simulink model "model_sim_CHB5_36pulse_23b"  (R2023b)
settings: Solver=FixedStepAuto  StartTime=0.0  StopTime=10  RelTol=1e-3
InitFcn:
  | sysinit
values from neighbouring files (symbols this model uses):
  C = 0.03    [sysinit.m]
  C_f = 0.625e-6    (= 6.25e-07)    [sysinit.m]
  L = 0.004    [sysinit.m]
  L_f = 3e-6    (= 3e-06)    [sysinit.m]
  R = 1.2    [sysinit.m]
  R_f = 1.5    [sysinit.m]
  st = 5e-7    (= 5e-07)    [sysinit.m]
libraries: spsSeriesRLCBranchLib x142, spsDiodeLib x60, spsIGBTLib x48, spsCurrentMeasurementLib x22, spsRMSLib x9, spsVoltageMeasurementLib x9, spsThreePhaseVIMeasurementLib x7, spsZigzagPhaseShiftingTransformerLib x6, spsUniversalBridgeLib x6, spsOnDelayLib x6, simulink x5, spsDistributedParametersLineLib x1
(part 3 of 3)

== system model_sim_CHB5_36pulse_23b/Subsystem/IGCT5 ==
  PWM : Inport
  Current Measurement1 : spsCurrentMeasurementLib/Current Measurement  PhasorSimulation=off  OutputType=Complex  PSBequivalent=0
  Demux : Demux
  Diode{1..3,6,8} (5 alike) : spsDiodeLib/Diode  Ron=DIODE.rF  Lon=0  Vf=DIODE.VF0  IC=0  UseSnubber=off  Rs=500  Cs=250e-9  Measurements=on
  IGBT{,1..3} (4 alike) : spsIGBTLib/IGBT  Ron=IGCT.rT  Lon=0  Vf=IGCT.VT0  Tf=1e-6  Tt=2e-6  IC=0  Rs=1e5  Cs=inf  Measurements=on
  Series RLC Branch1 : spsSeriesRLCBranchLib/Series RLC Branch  LConnTagsString=__new0  RConnTagsString=__new0  BranchType=RL  Resistance=1e-5  Inductance=3.0E-6  SetiL0=off  InitialCurrent=0  Capacitance=1e-6  Setx0=off  InitialVoltage=0  Measurements=None
  Series RLC Branch10 : spsSeriesRLCBranchLib/Series RLC Branch  LConnTagsString=__new0  RConnTagsString=__new0  BranchType=L  Resistance=1  Inductance=0.4e-6  SetiL0=off  InitialCurrent=0  Capacitance=1e-6  Setx0=off  InitialVoltage=0  Measurements=None
  Series RLC Branch12 : spsSeriesRLCBranchLib/Series RLC Branch  LConnTagsString=__new0  RConnTagsString=__new0  BranchType=RL  Resistance=1e-5  Inductance=1E-9  SetiL0=off  InitialCurrent=0  Capacitance=1e-6  Setx0=off  InitialVoltage=0  Measurements=None
  Series RLC Branch14 : spsSeriesRLCBranchLib/Series RLC Branch  LConnTagsString=__new0  RConnTagsString=__new0  BranchType=L  Resistance=1  Inductance=1E-7  SetiL0=off  InitialCurrent=0  Capacitance=1e-6  Setx0=off  InitialVoltage=0  Measurements=None
  Series RLC Branch2 : spsSeriesRLCBranchLib/Series RLC Branch  LConnTagsString=__new0  RConnTagsString=__new0  BranchType=RC  Resistance=1e-5  Inductance=20e-6  SetiL0=off  InitialCurrent=0  Capacitance=17e-6  Setx0=off  InitialVoltage=0  Measurements=None
  Series RLC Branch3 : spsSeriesRLCBranchLib/Series RLC Branch  LConnTagsString=__new0  RConnTagsString=__new0  BranchType=RL  Resistance=1e-5  Inductance=1E-9  SetiL0=off  InitialCurrent=0  Capacitance=1e-6  Setx0=off  InitialVoltage=0  Measurements=None
  Series RLC Branch5 : spsSeriesRLCBranchLib/Series RLC Branch  LConnTagsString=__new0  RConnTagsString=__new0  BranchType=L  Resistance=1  Inductance=1E-7  SetiL0=off  InitialCurrent=0  Capacitance=1e-6  Setx0=off  InitialVoltage=0  Measurements=None
  Series RLC Branch7 : spsSeriesRLCBranchLib/Series RLC Branch  LConnTagsString=__new0  RConnTagsString=__new0  BranchType=RL  Resistance=0.6  Inductance=1e-6  SetiL0=off  InitialCurrent=0  Capacitance=1e-6  Setx0=off  InitialVoltage=0  Measurements=None
  Series RLC Branch9 : spsSeriesRLCBranchLib/Series RLC Branch  LConnTagsString=__new0  RConnTagsString=__new0  BranchType=L  Resistance=1  Inductance=0.4e-6  SetiL0=off  InitialCurrent=0  Capacitance=1e-6  Setx0=off  InitialVoltage=0  Measurements=None
  Terminator{,1..9} (10 alike) : Terminator
  Udc+ : PMIOPort  Side=Left
  udc- : PMIOPort  Port=2  Side=Left
  p1 : PMIOPort  Port=3  Side=Right
  p2 : PMIOPort  Port=4  Side=Right
  wires:
  Diode3/1 -> Terminator9/1
  IGBT3/1 -> Terminator5/1
  [n1] -> IGBT3/1
  IGBT1/1 -> Terminator4/1
  IGBT2/1 -> Terminator3/1
  IGBT/1 -> Terminator2/1
  [n2] -> IGBT1/1
  [p1] -> IGBT2/1
  Current Measurement1/1 -> Terminator/1
  Diode2/1 -> Terminator8/1
  [p2] -> IGBT/1
  Diode8/1 -> Terminator7/1
  Diode1/1 -> Terminator6/1
  Diode6/1 -> Terminator1/1
  Demux/3 -> [n2]
  PWM/1 -> Demux/1
  Demux/1 -> [p2]
  Demux/2 -> [p1]
  Demux/4 -> [n1]
  connections:
  Series RLC Branch10/LConn1 -- udc-/RConn1
  Series RLC Branch9/LConn1 -- Udc+/RConn1
  Diode6/RConn1 -- Series RLC Branch7/RConn1 -- Series RLC Branch2/LConn1
  Current Measurement1/LConn1 -- Series RLC Branch1/RConn1 -- Series RLC Branch3/LConn1 -- Series RLC Branch12/LConn1
  IGBT3/RConn1 -- Series RLC Branch14/RConn1 -- Diode3/LConn1
  Series RLC Branch3/RConn1 -- IGBT/LConn1 -- Diode8/RConn1
  IGBT1/RConn1 -- Series RLC Branch5/RConn1 -- Diode1/LConn1
  Current Measurement1/RConn1 -- Diode6/LConn1
  Diode2/RConn1 -- Series RLC Branch12/RConn1 -- IGBT2/LConn1
  Diode2/LConn1 -- p1/RConn1 -- IGBT3/LConn1 -- IGBT2/RConn1 -- Diode3/RConn1
  Series RLC Branch5/LConn1 -- Series RLC Branch14/LConn1 -- Series RLC Branch10/RConn1 -- Series RLC Branch2/RConn1
  Series RLC Branch1/LConn1 -- Series RLC Branch7/LConn1 -- Series RLC Branch9/RConn1
  IGBT1/LConn1 -- p2/RConn1 -- Diode8/LConn1 -- IGBT/RConn1 -- Diode1/RConn1

== system model_sim_CHB5_36pulse_23b/Subsystem/IGCT6 ==
  PWM : Inport
  Current Measurement1 : spsCurrentMeasurementLib/Current Measurement  PhasorSimulation=off  OutputType=Complex  PSBequivalent=0
  Demux : Demux
  Diode{1..3,6,8} (5 alike) : spsDiodeLib/Diode  Ron=DIODE.rF  Lon=0  Vf=DIODE.VF0  IC=0  UseSnubber=off  Rs=500  Cs=250e-9  Measurements=on
  IGBT{,1..3} (4 alike) : spsIGBTLib/IGBT  Ron=IGCT.rT  Lon=0  Vf=IGCT.VT0  Tf=1e-6  Tt=2e-6  IC=0  Rs=1e5  Cs=inf  Measurements=on
  Series RLC Branch1 : spsSeriesRLCBranchLib/Series RLC Branch  LConnTagsString=__new0  RConnTagsString=__new0  BranchType=RL  Resistance=1e-5  Inductance=3.0E-6  SetiL0=off  InitialCurrent=0  Capacitance=1e-6  Setx0=off  InitialVoltage=0  Measurements=None
  Series RLC Branch10 : spsSeriesRLCBranchLib/Series RLC Branch  LConnTagsString=__new0  RConnTagsString=__new0  BranchType=L  Resistance=1  Inductance=0.4e-6  SetiL0=off  InitialCurrent=0  Capacitance=1e-6  Setx0=off  InitialVoltage=0  Measurements=None
  Series RLC Branch12 : spsSeriesRLCBranchLib/Series RLC Branch  LConnTagsString=__new0  RConnTagsString=__new0  BranchType=RL  Resistance=1e-5  Inductance=1E-9  SetiL0=off  InitialCurrent=0  Capacitance=1e-6  Setx0=off  InitialVoltage=0  Measurements=None
  Series RLC Branch14 : spsSeriesRLCBranchLib/Series RLC Branch  LConnTagsString=__new0  RConnTagsString=__new0  BranchType=L  Resistance=1  Inductance=1E-7  SetiL0=off  InitialCurrent=0  Capacitance=1e-6  Setx0=off  InitialVoltage=0  Measurements=None
  Series RLC Branch2 : spsSeriesRLCBranchLib/Series RLC Branch  LConnTagsString=__new0  RConnTagsString=__new0  BranchType=RC  Resistance=1e-5  Inductance=20e-6  SetiL0=off  InitialCurrent=0  Capacitance=17e-6  Setx0=off  InitialVoltage=0  Measurements=None
  Series RLC Branch3 : spsSeriesRLCBranchLib/Series RLC Branch  LConnTagsString=__new0  RConnTagsString=__new0  BranchType=RL  Resistance=1e-5  Inductance=1E-9  SetiL0=off  InitialCurrent=0  Capacitance=1e-6  Setx0=off  InitialVoltage=0  Measurements=None
  Series RLC Branch5 : spsSeriesRLCBranchLib/Series RLC Branch  LConnTagsString=__new0  RConnTagsString=__new0  BranchType=L  Resistance=1  Inductance=1E-7  SetiL0=off  InitialCurrent=0  Capacitance=1e-6  Setx0=off  InitialVoltage=0  Measurements=None
  Series RLC Branch7 : spsSeriesRLCBranchLib/Series RLC Branch  LConnTagsString=__new0  RConnTagsString=__new0  BranchType=RL  Resistance=0.6  Inductance=1e-6  SetiL0=off  InitialCurrent=0  Capacitance=1e-6  Setx0=off  InitialVoltage=0  Measurements=None
  Series RLC Branch9 : spsSeriesRLCBranchLib/Series RLC Branch  LConnTagsString=__new0  RConnTagsString=__new0  BranchType=L  Resistance=1  Inductance=0.4e-6  SetiL0=off  InitialCurrent=0  Capacitance=1e-6  Setx0=off  InitialVoltage=0  Measurements=None
  Terminator{,1..9} (10 alike) : Terminator
  Udc+ : PMIOPort  Side=Left
  udc- : PMIOPort  Port=2  Side=Left
  p1 : PMIOPort  Port=3  Side=Right
  p2 : PMIOPort  Port=4  Side=Right
  wires:
  Demux/4 -> [n1]
  Demux/2 -> [p1]
  Demux/1 -> [p2]
  PWM/1 -> Demux/1
  Demux/3 -> [n2]
  Diode6/1 -> Terminator1/1
  Diode1/1 -> Terminator6/1
  Diode8/1 -> Terminator7/1
  [p2] -> IGBT/1
  Diode2/1 -> Terminator8/1
  Current Measurement1/1 -> Terminator/1
  [p1] -> IGBT2/1
  [n2] -> IGBT1/1
  IGBT/1 -> Terminator2/1
  IGBT2/1 -> Terminator3/1
  IGBT1/1 -> Terminator4/1
  [n1] -> IGBT3/1
  IGBT3/1 -> Terminator5/1
  Diode3/1 -> Terminator9/1
  connections:
  Diode1/RConn1 -- IGBT/RConn1 -- Diode8/LConn1 -- p2/RConn1 -- IGBT1/LConn1
  Series RLC Branch9/RConn1 -- Series RLC Branch7/LConn1 -- Series RLC Branch1/LConn1
  Series RLC Branch2/RConn1 -- Series RLC Branch10/RConn1 -- Series RLC Branch14/LConn1 -- Series RLC Branch5/LConn1
  Diode3/RConn1 -- IGBT2/RConn1 -- IGBT3/LConn1 -- p1/RConn1 -- Diode2/LConn1
  IGBT2/LConn1 -- Series RLC Branch12/RConn1 -- Diode2/RConn1
  Current Measurement1/RConn1 -- Diode6/LConn1
  Diode1/LConn1 -- Series RLC Branch5/RConn1 -- IGBT1/RConn1
  Diode8/RConn1 -- IGBT/LConn1 -- Series RLC Branch3/RConn1
  Diode3/LConn1 -- Series RLC Branch14/RConn1 -- IGBT3/RConn1
  Series RLC Branch12/LConn1 -- Series RLC Branch3/LConn1 -- Series RLC Branch1/RConn1 -- Current Measurement1/LConn1
  Series RLC Branch2/LConn1 -- Series RLC Branch7/RConn1 -- Diode6/RConn1
  Series RLC Branch9/LConn1 -- Udc+/RConn1
  Series RLC Branch10/LConn1 -- udc-/RConn1

== system model_sim_CHB5_36pulse_23b/Uref/Saddle_Wave ==
  A : Inport
  B : Inport  Port=2
  C : Inport  Port=3
  Add{1..3,9} (4 alike) : Sum
  Gain : Gain  Gain=-0.5
  Max : MinMax  Function=max  Inputs=3
  Max1 : MinMax  Inputs=3
  a : Outport
  b : Outport  Port=2
  c : Outport  Port=3
  wires:
  B/1 -> Add3/2, Max1/2, Max/2
  C/1 -> Add9/2, Max1/3, Max/3
  A/1 -> Max1/1, Add2/2, Max/1
  Gain/1 -> Add9/1, Add3/1, Add2/1
  Max/1 -> Add1/1
  Max1/1 -> Add1/2
  Add1/1 -> Gain/1
  Add9/1 -> c/1
  Add2/1 -> a/1
  Add3/1 -> b/1

== system model_sim_CHB5_36pulse_23b/pwm generator/PD ==
  Mux2 : Mux
  Repeating Sequence1 : simulink/Sources/Repeating Sequence  rep_seq_t=[0 0.5 1]*(1/f_car)  rep_seq_y=[0 1 0]*500
  Repeating Sequence2 : simulink/Sources/Repeating Sequence  rep_seq_t=[0 0.5 1]*(1/f_car)  rep_seq_y=[-2 -1 -2]*500
  Repeating Sequence3 : simulink/Sources/Repeating Sequence  rep_seq_t=[0 0.5 1]*(1/f_car)  rep_seq_y=[1 2 1]*500
  Repeating Sequence4 : simulink/Sources/Repeating Sequence  rep_seq_t=[0 0.5 1]*(1/f_car)  rep_seq_y=[-1 0 -1]*500
  carrier_4*1 : Outport
  wires:
  Repeating Sequence2/1 -> Mux2/4
  Mux2/1 -> carrier_4*1/1  "carrier_4*1"
  Repeating Sequence3/1 -> Mux2/1
  Repeating Sequence4/1 -> Mux2/3
  Repeating Sequence1/1 -> Mux2/2

== system model_sim_CHB5_36pulse_23b/pwm generator/Subsystem ==
  modulate_wave : Inport
  Carrier_wave : Inport  Port=2
  Demux1 : Demux
  Logical Operator{1..4} (4 alike) : Logic  Operator=NOT  AllPortsSameDT=off  OutDataTypeStr=boolean
  Mux : Mux
  Mux1 : Mux
  Relational Operator2 : RelationalOperator  Operator=>  OutDataTypeStr=boolean  RndMeth=Simplest  InputSameDT=off
  Relational Operator3 : RelationalOperator  Operator=>  OutDataTypeStr=boolean  RndMeth=Simplest  InputSameDT=off
  Relational Operator4 : RelationalOperator  Operator=<  OutDataTypeStr=boolean  RndMeth=Simplest  InputSameDT=off
  Relational Operator5 : RelationalOperator  Operator=<  OutDataTypeStr=boolean  RndMeth=Simplest  InputSameDT=off
  pwm_up : Outport
  pwm_down : Outport  Port=2
  wires:
  Demux1/1 -> Relational Operator2/2
  Relational Operator5/1 -> Mux1/2, Logical Operator3/1
  Logical Operator2/1 -> Mux/4
  modulate_wave/1 -> Relational Operator5/1, Relational Operator4/1, Relational Operator3/1, Relational Operator2/1
  Demux1/4 -> Relational Operator5/2
  Demux1/2 -> Relational Operator3/2
  Demux1/3 -> Relational Operator4/2
  Logical Operator4/1 -> Mux/3
  Relational Operator4/1 -> Mux/2, Logical Operator2/1
  Relational Operator2/1 -> Mux/1, Logical Operator4/1
  Logical Operator1/1 -> Mux1/3
  Relational Operator3/1 -> Mux1/1, Logical Operator1/1
  Logical Operator3/1 -> Mux1/4
  Carrier_wave/1 -> Demux1/1
  Mux/1 -> pwm_up/1  "pwm_up"
  Mux1/1 -> pwm_down/1  "pwm_down"

== system model_sim_CHB5_36pulse_23b/pwm generator/Subsystem1 ==
  modulate_wave : Inport
  Carrier_wave : Inport  Port=2
  Demux1 : Demux
  Logical Operator{1..4} (4 alike) : Logic  Operator=NOT  AllPortsSameDT=off  OutDataTypeStr=boolean
  Mux : Mux
  Mux1 : Mux
  Relational Operator2 : RelationalOperator  Operator=>  OutDataTypeStr=boolean  RndMeth=Simplest  InputSameDT=off
  Relational Operator3 : RelationalOperator  Operator=>  OutDataTypeStr=boolean  RndMeth=Simplest  InputSameDT=off
  Relational Operator4 : RelationalOperator  Operator=<  OutDataTypeStr=boolean  RndMeth=Simplest  InputSameDT=off
  Relational Operator5 : RelationalOperator  Operator=<  OutDataTypeStr=boolean  RndMeth=Simplest  InputSameDT=off
  pwm_up : Outport
  pwm_down : Outport  Port=2
  wires:
  Mux1/1 -> pwm_down/1  "pwm_down"
  Mux/1 -> pwm_up/1  "pwm_up"
  Carrier_wave/1 -> Demux1/1
  Logical Operator3/1 -> Mux1/4
  Relational Operator3/1 -> Logical Operator1/1, Mux1/1
  Logical Operator1/1 -> Mux1/3
  Relational Operator2/1 -> Logical Operator4/1, Mux/1
  Relational Operator4/1 -> Logical Operator2/1, Mux/2
  Logical Operator4/1 -> Mux/3
  Demux1/3 -> Relational Operator4/2
  Demux1/2 -> Relational Operator3/2
  Demux1/4 -> Relational Operator5/2
  modulate_wave/1 -> Relational Operator2/1, Relational Operator3/1, Relational Operator4/1, Relational Operator5/1
  Logical Operator2/1 -> Mux/4
  Relational Operator5/1 -> Logical Operator3/1, Mux1/2
  Demux1/1 -> Relational Operator2/2

== system model_sim_CHB5_36pulse_23b/pwm generator/Subsystem2 ==
  modulate_wave : Inport
  Carrier_wave : Inport  Port=2
  Demux1 : Demux
  Logical Operator{1..4} (4 alike) : Logic  Operator=NOT  AllPortsSameDT=off  OutDataTypeStr=boolean
  Mux : Mux
  Mux1 : Mux
  Relational Operator2 : RelationalOperator  Operator=>  OutDataTypeStr=boolean  RndMeth=Simplest  InputSameDT=off
  Relational Operator3 : RelationalOperator  Operator=>  OutDataTypeStr=boolean  RndMeth=Simplest  InputSameDT=off
  Relational Operator4 : RelationalOperator  Operator=<  OutDataTypeStr=boolean  RndMeth=Simplest  InputSameDT=off
  Relational Operator5 : RelationalOperator  Operator=<  OutDataTypeStr=boolean  RndMeth=Simplest  InputSameDT=off
  pwm_up : Outport
  pwm_down : Outport  Port=2
  wires:
  Demux1/1 -> Relational Operator2/2
  Relational Operator5/1 -> Mux1/2, Logical Operator3/1
  Logical Operator2/1 -> Mux/4
  modulate_wave/1 -> Relational Operator5/1, Relational Operator4/1, Relational Operator3/1, Relational Operator2/1
  Demux1/4 -> Relational Operator5/2
  Demux1/2 -> Relational Operator3/2
  Demux1/3 -> Relational Operator4/2
  Logical Operator4/1 -> Mux/3
  Relational Operator4/1 -> Mux/2, Logical Operator2/1
  Relational Operator2/1 -> Mux/1, Logical Operator4/1
  Logical Operator1/1 -> Mux1/3
  Relational Operator3/1 -> Mux1/1, Logical Operator1/1
  Logical Operator3/1 -> Mux1/4
  Carrier_wave/1 -> Demux1/1
  Mux/1 -> pwm_up/1  "pwm_up"
  Mux1/1 -> pwm_down/1  "pwm_down"

== system model_sim_CHB5_36pulse_23b/pwm generator/carrier1 ==
  Mux : Mux
  Repeating Sequence1 : simulink/Sources/Repeating Sequence  rep_seq_t=[0 0.5 1]/f_car  rep_seq_y=[-1 1 -1]*1000
  Scope1 : Scope  NumInputPorts=4
  Transport Delay1 : TransportDelay  DelayTime=tt/f_car  BufferSize=3072
  Transport Delay3 : TransportDelay  DelayTime=tt/f_car  BufferSize=3072
  Transport Delay4 : TransportDelay  DelayTime=tt/f_car  BufferSize=3072
  CARRIER_4*1 : Outport
  wires:
  Repeating Sequence1/1 -> Scope1/1, Mux/1, Transport Delay1/1
  Transport Delay1/1 -> Scope1/2, Mux/2, Transport Delay3/1
  Mux/1 -> CARRIER_4*1/1
  Transport Delay3/1 -> Mux/3, Scope1/3, Transport Delay4/1
  Transport Delay4/1 -> Mux/4, Scope1/4

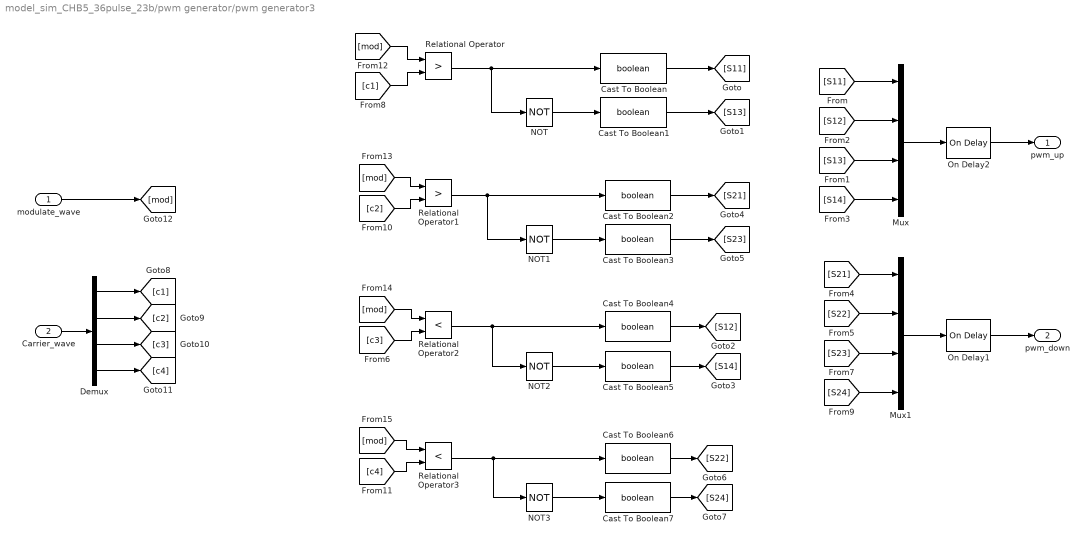
== system model_sim_CHB5_36pulse_23b/pwm generator/pwm generator3 ==
  modulate_wave : Inport
  Carrier_wave : Inport  Port=2
  Cast To Boolean{,1..7} (8 alike) : DataTypeConversion  OutDataTypeStr=boolean  SaturateOnIntegerOverflow=off  RndMeth=Floor
  Demux : Demux
  Mux : Mux
  Mux1 : Mux
  NOT{,1..3} (4 alike) : Logic  Operator=NOT  AllPortsSameDT=off  OutDataTypeStr=boolean
  On Delay1 : spsOnDelayLib/On Delay  DelayType=On delay  delay=ttd  ic=0  Ts=0
  On Delay2 : spsOnDelayLib/On Delay  DelayType=On delay  delay=ttd  ic=0  Ts=0
  Relational Operator : RelationalOperator  Operator=>  OutDataTypeStr=boolean  RndMeth=Simplest  InputSameDT=off
  Relational Operator1 : RelationalOperator  Operator=>  OutDataTypeStr=boolean  RndMeth=Simplest  InputSameDT=off
  Relational Operator2 : RelationalOperator  Operator=<  OutDataTypeStr=boolean  RndMeth=Simplest  InputSameDT=off
  Relational Operator3 : RelationalOperator  Operator=<  OutDataTypeStr=boolean  RndMeth=Simplest  InputSameDT=off
  pwm_up : Outport
  pwm_down : Outport  Port=2
  wires:
  NOT/1 -> Cast To Boolean1/1
  [S14] -> Mux/4
  [S23] -> Mux1/3
  [S12] -> Mux/2
  NOT2/1 -> Cast To Boolean5/1
  [S21] -> Mux1/1
  Relational Operator1/1 -> NOT1/1, Cast To Boolean2/1
  [S22] -> Mux1/2
  NOT3/1 -> Cast To Boolean7/1
  Mux/1 -> On Delay2/1
  [S24] -> Mux1/4
  [S13] -> Mux/3
  Relational Operator2/1 -> Cast To Boolean4/1, NOT2/1
  [S11] -> Mux/1
  Relational Operator/1 -> NOT/1, Cast To Boolean/1
  NOT1/1 -> Cast To Boolean3/1
  Mux1/1 -> On Delay1/1
  Relational Operator3/1 -> Cast To Boolean6/1, NOT3/1
  On Delay1/1 -> pwm_down/1
  On Delay2/1 -> pwm_up/1
  Cast To Boolean/1 -> [S11]
  Cast To Boolean1/1 -> [S13]
  Cast To Boolean2/1 -> [S21]
  Cast To Boolean3/1 -> [S23]
  Cast To Boolean4/1 -> [S12]
  Cast To Boolean5/1 -> [S14]
  Cast To Boolean6/1 -> [S22]
  Cast To Boolean7/1 -> [S24]
  Carrier_wave/1 -> Demux/1
  Demux/1 -> [c1]
  [c3] -> Relational Operator2/2
  Demux/2 -> [c2]
  Demux/4 -> [c4]
  Demux/3 -> [c3]
  [c1] -> Relational Operator/2
  [c2] -> Relational Operator1/2
  [c4] -> Relational Operator3/2
  modulate_wave/1 -> [mod]
  [mod] -> Relational Operator/1
  [mod] -> Relational Operator3/1
  [mod] -> Relational Operator2/1
  [mod] -> Relational Operator1/1

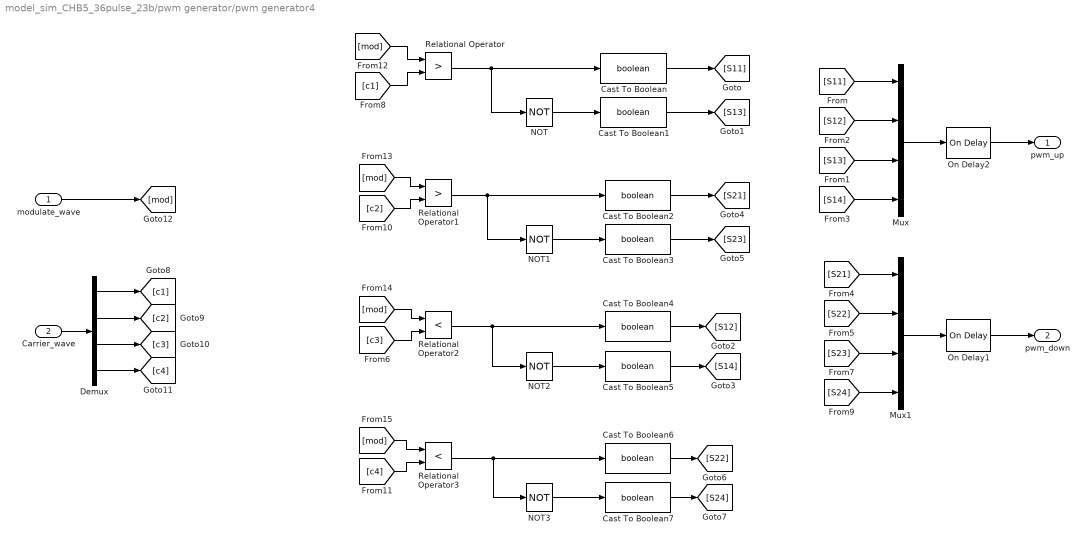
== system model_sim_CHB5_36pulse_23b/pwm generator/pwm generator4 ==
  modulate_wave : Inport
  Carrier_wave : Inport  Port=2
  Cast To Boolean{,1..7} (8 alike) : DataTypeConversion  OutDataTypeStr=boolean  SaturateOnIntegerOverflow=off  RndMeth=Floor
  Demux : Demux
  Mux : Mux
  Mux1 : Mux
  NOT{,1..3} (4 alike) : Logic  Operator=NOT  AllPortsSameDT=off  OutDataTypeStr=boolean
  On Delay1 : spsOnDelayLib/On Delay  DelayType=On delay  delay=ttd  ic=0  Ts=0
  On Delay2 : spsOnDelayLib/On Delay  DelayType=On delay  delay=ttd  ic=0  Ts=0
  Relational Operator : RelationalOperator  Operator=>  OutDataTypeStr=boolean  RndMeth=Simplest  InputSameDT=off
  Relational Operator1 : RelationalOperator  Operator=>  OutDataTypeStr=boolean  RndMeth=Simplest  InputSameDT=off
  Relational Operator2 : RelationalOperator  Operator=<  OutDataTypeStr=boolean  RndMeth=Simplest  InputSameDT=off
  Relational Operator3 : RelationalOperator  Operator=<  OutDataTypeStr=boolean  RndMeth=Simplest  InputSameDT=off
  pwm_up : Outport
  pwm_down : Outport  Port=2
  wires:
  [mod] -> Relational Operator1/1
  [mod] -> Relational Operator2/1
  [mod] -> Relational Operator3/1
  [mod] -> Relational Operator/1
  modulate_wave/1 -> [mod]
  [c4] -> Relational Operator3/2
  [c2] -> Relational Operator1/2
  [c1] -> Relational Operator/2
  Demux/3 -> [c3]
  Demux/4 -> [c4]
  Demux/2 -> [c2]
  [c3] -> Relational Operator2/2
  Demux/1 -> [c1]
  Carrier_wave/1 -> Demux/1
  Cast To Boolean7/1 -> [S24]
  Cast To Boolean6/1 -> [S22]
  Cast To Boolean5/1 -> [S14]
  Cast To Boolean4/1 -> [S12]
  Cast To Boolean3/1 -> [S23]
  Cast To Boolean2/1 -> [S21]
  Cast To Boolean1/1 -> [S13]
  Cast To Boolean/1 -> [S11]
  On Delay2/1 -> pwm_up/1
  On Delay1/1 -> pwm_down/1
  Relational Operator3/1 -> NOT3/1, Cast To Boolean6/1
  Mux1/1 -> On Delay1/1
  NOT1/1 -> Cast To Boolean3/1
  Relational Operator/1 -> Cast To Boolean/1, NOT/1
  [S11] -> Mux/1
  Relational Operator2/1 -> NOT2/1, Cast To Boolean4/1
  [S13] -> Mux/3
  [S24] -> Mux1/4
  Mux/1 -> On Delay2/1
  NOT3/1 -> Cast To Boolean7/1
  [S22] -> Mux1/2
  Relational Operator1/1 -> Cast To Boolean2/1, NOT1/1
  [S21] -> Mux1/1
  NOT2/1 -> Cast To Boolean5/1
  [S12] -> Mux/2
  [S23] -> Mux1/3
  [S14] -> Mux/4
  NOT/1 -> Cast To Boolean1/1

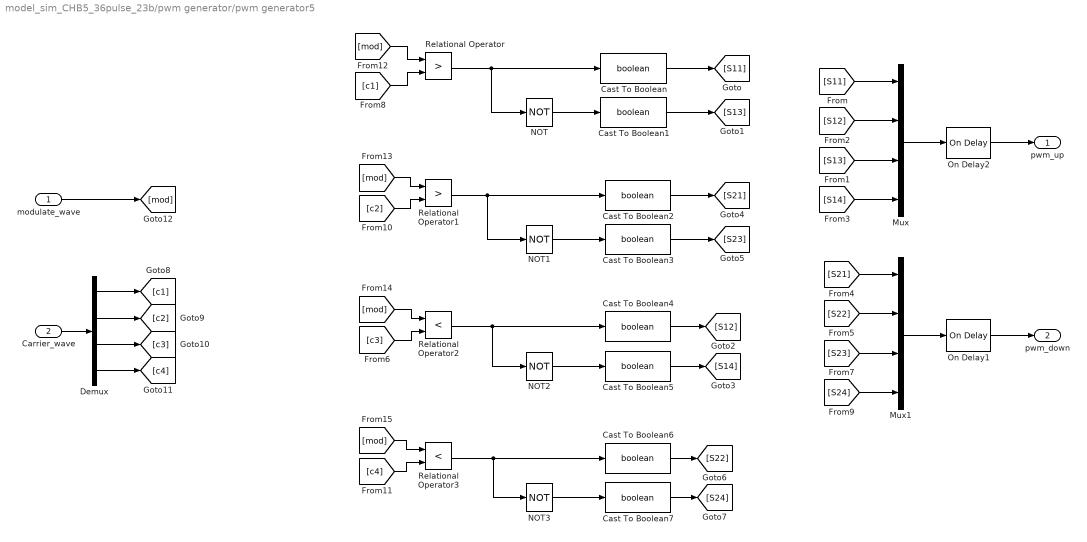
== system model_sim_CHB5_36pulse_23b/pwm generator/pwm generator5 ==
  modulate_wave : Inport
  Carrier_wave : Inport  Port=2
  Cast To Boolean{,1..7} (8 alike) : DataTypeConversion  OutDataTypeStr=boolean  SaturateOnIntegerOverflow=off  RndMeth=Floor
  Demux : Demux
  Mux : Mux
  Mux1 : Mux
  NOT{,1..3} (4 alike) : Logic  Operator=NOT  AllPortsSameDT=off  OutDataTypeStr=boolean
  On Delay1 : spsOnDelayLib/On Delay  DelayType=On delay  delay=ttd  ic=0  Ts=0
  On Delay2 : spsOnDelayLib/On Delay  DelayType=On delay  delay=ttd  ic=0  Ts=0
  Relational Operator : RelationalOperator  Operator=>  OutDataTypeStr=boolean  RndMeth=Simplest  InputSameDT=off
  Relational Operator1 : RelationalOperator  Operator=>  OutDataTypeStr=boolean  RndMeth=Simplest  InputSameDT=off
  Relational Operator2 : RelationalOperator  Operator=<  OutDataTypeStr=boolean  RndMeth=Simplest  InputSameDT=off
  Relational Operator3 : RelationalOperator  Operator=<  OutDataTypeStr=boolean  RndMeth=Simplest  InputSameDT=off
  pwm_up : Outport
  pwm_down : Outport  Port=2
  wires:
  NOT/1 -> Cast To Boolean1/1
  [S14] -> Mux/4
  [S23] -> Mux1/3
  [S12] -> Mux/2
  NOT2/1 -> Cast To Boolean5/1
  [S21] -> Mux1/1
  Relational Operator1/1 -> NOT1/1, Cast To Boolean2/1
  [S22] -> Mux1/2
  NOT3/1 -> Cast To Boolean7/1
  Mux/1 -> On Delay2/1
  [S24] -> Mux1/4
  [S13] -> Mux/3
  Relational Operator2/1 -> Cast To Boolean4/1, NOT2/1
  [S11] -> Mux/1
  Relational Operator/1 -> NOT/1, Cast To Boolean/1
  NOT1/1 -> Cast To Boolean3/1
  Mux1/1 -> On Delay1/1
  Relational Operator3/1 -> Cast To Boolean6/1, NOT3/1
  On Delay1/1 -> pwm_down/1
  On Delay2/1 -> pwm_up/1
  Cast To Boolean/1 -> [S11]
  Cast To Boolean1/1 -> [S13]
  Cast To Boolean2/1 -> [S21]
  Cast To Boolean3/1 -> [S23]
  Cast To Boolean4/1 -> [S12]
  Cast To Boolean5/1 -> [S14]
  Cast To Boolean6/1 -> [S22]
  Cast To Boolean7/1 -> [S24]
  Carrier_wave/1 -> Demux/1
  Demux/1 -> [c1]
  [c3] -> Relational Operator2/2
  Demux/2 -> [c2]
  Demux/4 -> [c4]
  Demux/3 -> [c3]
  [c1] -> Relational Operator/2
  [c2] -> Relational Operator1/2
  [c4] -> Relational Operator3/2
  modulate_wave/1 -> [mod]
  [mod] -> Relational Operator/1
  [mod] -> Relational Operator3/1
  [mod] -> Relational Operator2/1
  [mod] -> Relational Operator1/1

== matlab function model_sim_CHB5_36pulse_23b/MATLAB Function ==
  data: u input; y output; i input
function y = fcn(u,i)

y =1.732*u*i;
